simulink model "autoland"  (Simulink 7.4)
settings: Solver=ode45  StartTime=0.0  StopTime=1000  RelTol=1e-3
libraries: simulink x3
settings Model: Creator=s139453  LastModifiedBy=Shihan Tissera
settings DebuggingCC: StrictBusMsg=ErrorLevel1

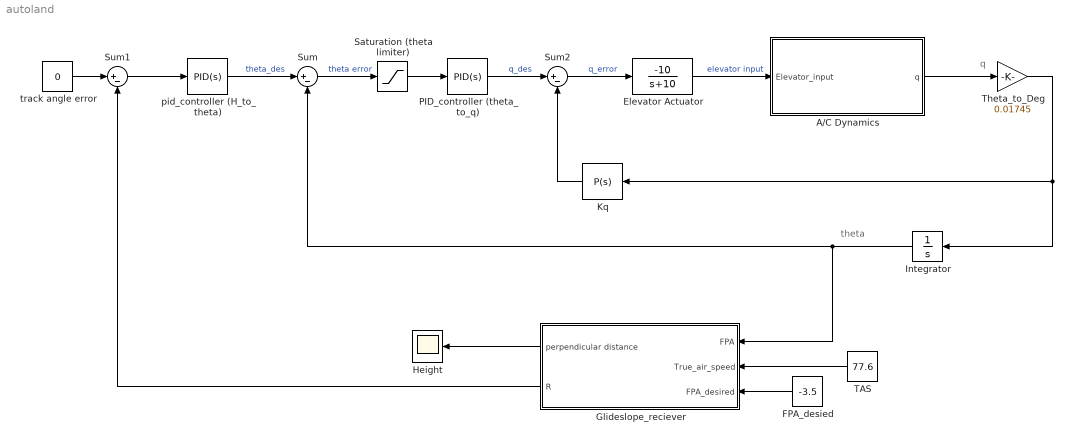
== system autoland ==
  note: q
  note: theta
  A/C Dynamics : Subsystem
  Elevator Actuator : TransferFcn  Numerator=-10  Denominator=[ 1 10]
  FPA_desied : Constant  Value=-3.5  OutDataType=fixdt(1, 16)  OutScaling=2^0
  Glideslope_reciever : Subsystem
  Height : Scope
  Integrator : Integrator
  Kq : simulink/Continuous/PID Controller  DialogController=pidpack.PIDConfig.pidDDGCreate  DialogControllerArgs=DataTag0  SystemSampleTime=-1  Controller=P  TimeDomain=Continuous-time  SampleTime=1  IntegratorMethod=Forward Euler  FilterMethod=Forward Euler  Form=Parallel  P=247.439962192662  I=0.613531573151948  D=-3.88575127512768  N=2.14186820429126  InitialConditionSource=internal  InitialConditionForIntegrator=0  InitialConditionForFilter=0  ExternalReset=none  LimitOutput=off  UpperSaturationLimit=inf  LowerSaturationLimit=-inf  LinearizeAsGain=off  AntiWindupMode=none  Kb=1  TrackingMode=off  Kt=1  PParamMin=[]  PParamMax=[]  IParamMin=[]  IParamMax=[]  DParamMin=[]  DParamMax=[]  NParamMin=[]  NParamMax=[]  KbParamMin=[]  KbParamMax=[]  KtParamMin=[]  KtParamMax=[]  POutMin=[]  POutMax=[]  IOutMin=[]  IOutMax=[]  DOutMin=[]  DOutMax=[]  NOutMin=[]  NOutMax=[]  KbOutMin=[]  KbOutMax=[]  KtOutMin=[]  KtOutMax=[]  IntegratorOutMin=[]  IntegratorOutMax=[]  FilterOutMin=[]  FilterOutMax=[]  SumOutMin=[]  SumOutMax=[]  SumI1OutMin=[]  SumI1OutMax=[]  SumI2OutMin=[]  SumI2OutMax=[]  SumI3OutMin=[]  SumI3OutMax=[]  SumDOutMin=[]  SumDOutMax=[]  SaturationOutMin=[]  SaturationOutMax=[]  IntegratorContinuousStateAttributes=''  IntegratorStateMustResolveToSignalObject=off  IntegratorRTWStateStorageClass=Auto  FilterContinuousStateAttributes=''  FilterStateMustResolveToSignalObject=off  FilterRTWStateStorageClass=Auto
  PID_controller (theta_to_q) : simulink/Continuous/PID Controller  DialogController=pidpack.PIDConfig.pidDDGCreate  DialogControllerArgs=DataTag1  SystemSampleTime=-1  Controller=PID  TimeDomain=Continuous-time  SampleTime=1  IntegratorMethod=Forward Euler  FilterMethod=Forward Euler  Form=Parallel  P=1244.9386840592  I=45.1749343460384  D=-205.781331416083  N=4.10064947727353  InitialConditionSource=internal  InitialConditionForIntegrator=0  InitialConditionForFilter=0  ExternalReset=none  LimitOutput=off  UpperSaturationLimit=inf  LowerSaturationLimit=-inf  LinearizeAsGain=off  AntiWindupMode=none  Kb=1  TrackingMode=off  Kt=1  PParamMin=[]  PParamMax=[]  IParamMin=[]  IParamMax=[]  DParamMin=[]  DParamMax=[]  NParamMin=[]  NParamMax=[]  KbParamMin=[]  KbParamMax=[]  KtParamMin=[]  KtParamMax=[]  POutMin=[]  POutMax=[]  IOutMin=[]  IOutMax=[]  DOutMin=[]  DOutMax=[]  NOutMin=[]  NOutMax=[]  KbOutMin=[]  KbOutMax=[]  KtOutMin=[]  KtOutMax=[]  IntegratorOutMin=[]  IntegratorOutMax=[]  FilterOutMin=[]  FilterOutMax=[]  SumOutMin=[]  SumOutMax=[]  SumI1OutMin=[]  SumI1OutMax=[]  SumI2OutMin=[]  SumI2OutMax=[]  SumI3OutMin=[]  SumI3OutMax=[]  SumDOutMin=[]  SumDOutMax=[]  SaturationOutMin=[]  SaturationOutMax=[]  IntegratorContinuousStateAttributes=''  IntegratorStateMustResolveToSignalObject=off  IntegratorRTWStateStorageClass=Auto  FilterContinuousStateAttributes=''  FilterStateMustResolveToSignalObject=off  FilterRTWStateStorageClass=Auto
  Saturation (theta limiter) : Saturate  UpperLimit=0.3  LowerLimit=-0.3
  Sum : Sum  Inputs=|+-
  Sum1 : Sum  Inputs=|+-  OutDataType=fixdt(1, 16)  OutScaling=2^0
  Sum2 : Sum  Inputs=|+-
  TAS : Constant  Value=77.6  OutDataType=fixdt(1, 16)  OutScaling=2^0
  Theta_to_Deg : Gain  Gain=0.01745  ParameterDataType=fixdt(1, 16)  ParameterScaling=2^0  OutDataType=fixdt(1, 16)  OutScaling=2^0
  pid_controller (H_to_theta) : simulink/Continuous/PID Controller  DialogController=pidpack.PIDConfig.pidDDGCreate  DialogControllerArgs=DataTag2  SystemSampleTime=-1  Controller=PID  TimeDomain=Continuous-time  SampleTime=1  IntegratorMethod=Forward Euler  FilterMethod=Forward Euler  Form=Parallel  P=0  I=-0.00335166989252525  D=0  N=100  InitialConditionSource=internal  InitialConditionForIntegrator=0  InitialConditionForFilter=0  ExternalReset=none  LimitOutput=off  UpperSaturationLimit=inf  LowerSaturationLimit=-inf  LinearizeAsGain=off  AntiWindupMode=none  Kb=1  TrackingMode=off  Kt=1  PParamMin=[]  PParamMax=[]  IParamMin=[]  IParamMax=[]  DParamMin=[]  DParamMax=[]  NParamMin=[]  NParamMax=[]  KbParamMin=[]  KbParamMax=[]  KtParamMin=[]  KtParamMax=[]  POutMin=[]  POutMax=[]  IOutMin=[]  IOutMax=[]  DOutMin=[]  DOutMax=[]  NOutMin=[]  NOutMax=[]  KbOutMin=[]  KbOutMax=[]  KtOutMin=[]  KtOutMax=[]  IntegratorOutMin=[]  IntegratorOutMax=[]  FilterOutMin=[]  FilterOutMax=[]  SumOutMin=[]  SumOutMax=[]  SumI1OutMin=[]  SumI1OutMax=[]  SumI2OutMin=[]  SumI2OutMax=[]  SumI3OutMin=[]  SumI3OutMax=[]  SumDOutMin=[]  SumDOutMax=[]  SaturationOutMin=[]  SaturationOutMax=[]  IntegratorContinuousStateAttributes=''  IntegratorStateMustResolveToSignalObject=off  IntegratorRTWStateStorageClass=Auto  FilterContinuousStateAttributes=''  FilterStateMustResolveToSignalObject=off  FilterRTWStateStorageClass=Auto
  track angle error : Constant  Value=0  OutDataType=fixdt(1, 16)  OutScaling=2^0
  wires:
  Elevator Actuator/1 -> A/C Dynamics/1(Elevator_input)  "elevator input"
  Integrator/1 -> Glideslope_reciever/1(FPA), Sum/2
  Sum2/1 -> Elevator Actuator/1  "q_error"
  Kq/1 -> Sum2/2
  Saturation (theta limiter)/1 -> PID_controller (theta_to_q)/1
  Sum/1 -> Saturation (theta limiter)/1  "theta error"
  A/C Dynamics/1(q) -> Theta_to_Deg/1
  Theta_to_Deg/1 -> Integrator/1, Kq/1
  PID_controller (theta_to_q)/1 -> Sum2/1  "q_des"
  pid_controller (H_to_theta)/1 -> Sum/1  "theta_des"
  Sum1/1 -> pid_controller (H_to_theta)/1
  track angle error/1 -> Sum1/1
  Glideslope_reciever/2(R) -> Sum1/2
  FPA_desied/1 -> Glideslope_reciever/3(FPA_desired)
  TAS/1 -> Glideslope_reciever/2(True_air_speed)
  Glideslope_reciever/1(perpendicular distance) -> Height/1

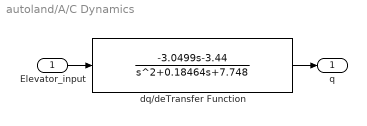
== system autoland/A/C Dynamics ==
  Elevator_input : Inport
  dq/deTransfer Function : TransferFcn  Numerator=[-3.0499 -3.44]  Denominator="[1  0.18464  7.748]"
  q : Outport
  wires:
  Elevator_input/1 -> dq/deTransfer Function/1
  dq/deTransfer Function/1 -> q/1

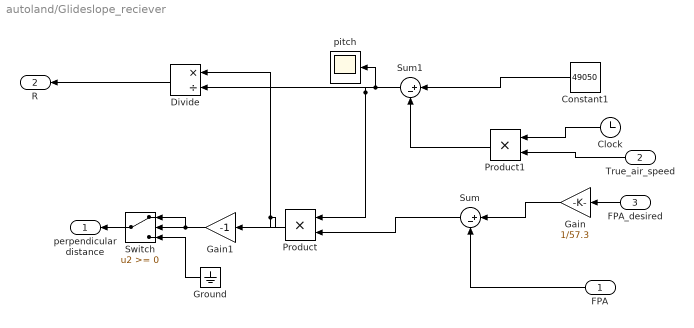
== system autoland/Glideslope_reciever ==
  FPA : Inport  OutDataType=fixdt(1, 16)  OutScaling=2^0
  True_air_speed : Inport  Port=2  OutDataType=fixdt(1, 16)  OutScaling=2^0
  FPA_desired : Inport  Port=3  OutDataType=fixdt(1, 16)  OutScaling=2^0
  Clock : Clock
      settings: Decimation=10
  Constant1 : Constant  Value=49050  OutDataType=fixdt(1, 16)  OutScaling=2^0
  Divide : Product  Inputs=*/  OutDataType=fixdt(1, 16)  OutScaling=2^-10
  Gain : Gain  Gain=1/57.3  ParameterDataType=fixdt(1, 16)  ParameterScaling=2^0  OutDataType=fixdt(1, 16)  OutScaling=2^0
  Gain1 : Gain  Gain=-1  ParameterDataType=fixdt(1, 16)  ParameterScaling=2^0  OutDataType=fixdt(1, 16)  OutScaling=2^0
  Ground : Ground
  Product : Product  OutDataType=fixdt(1, 16)  OutScaling=2^0  RndMeth=Zero
  Product1 : Product  OutDataType=fixdt(1, 16)  OutScaling=2^0  RndMeth=Zero
  Sum : Sum  Inputs=|+-  OutDataType=fixdt(1, 16)  OutScaling=2^0
  Sum1 : Sum  Inputs=|+-  OutDataType=fixdt(1, 16)  OutScaling=2^0
  Switch : Switch  OutDataType=fixdt(1, 16)  OutScaling=2^0
  pitch : Scope
      settings: SaveName=ScopeData3
  perpendicular distance : Outport  OutDataType=fixdt(1, 16)  OutScaling=2^0
  R : Outport  Port=2  OutDataType=fixdt(1, 16)  OutScaling=2^0
  wires:
  FPA_desired/1 -> Gain/1
  Gain/1 -> Sum/1
  FPA/1 -> Sum/2
  Clock/1 -> Product1/1
  True_air_speed/1 -> Product1/2
  Product1/1 -> Sum1/2
  Constant1/1 -> Sum1/1
  Sum/1 -> Product/2
  Sum1/1 -> Product/1, Divide/2, pitch/1
  Product/1 -> Divide/1, Gain1/1
  Divide/1 -> R/1
  Gain1/1 -> Switch/2, Switch/1
  Switch/1 -> perpendicular distance/1
  Ground/1 -> Switch/3
